simulink model "Spring_mass_damper_system"  (R2024a)
settings: Solver=VariableStepAuto  StartTime=0.0  StopTime=10  MaxStep=0.01  RelTol=1e-3
model workspace (MAT data in the model file):
  M = 10
  b = 50
  k = 100
settings Model: Creator=91839
settings SolverCC: AlgebraicLoopSolver=TrustRegion
settings DataIOCC: ExternalInput=data  LoadExternalInput=on  SaveFormat=Array  DSMLogging=off  ReturnWorkspaceOutputs=off
settings DebuggingCC: UnconnectedInputMsg=warning  UnconnectedOutputMsg=warning  UnconnectedLineMsg=warning
settings ModelReferenceCC: EnableRefExpFcnMdlSchedulingChecks=on
settings SFSimCC: CustomCodeUndefinedFunction=UseInterfaceOnly
settings RTWCC: GPUComputeCapability=3.5

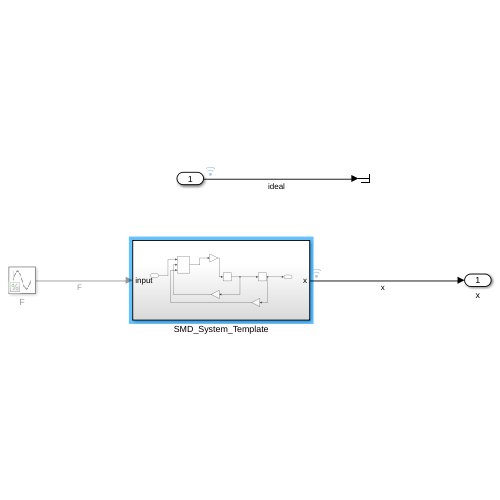
[thumbnail: Simulink's stored preview of the top-level diagram]
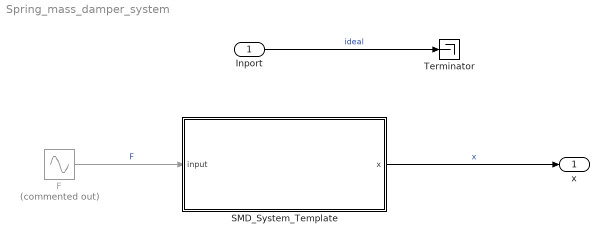
== system Spring_mass_damper_system ==
  Inport : Inport
  F : Sin  Commented=on  SampleTime=0
  SMD_System_Template : Subsystem
  Terminator : Terminator
  x : Outport
  wires:
  Inport/1 -> Terminator/1  "ideal"
  F/1 -> SMD_System_Template/1(input)  "F"
  SMD_System_Template/1(x) -> x/1  "x"

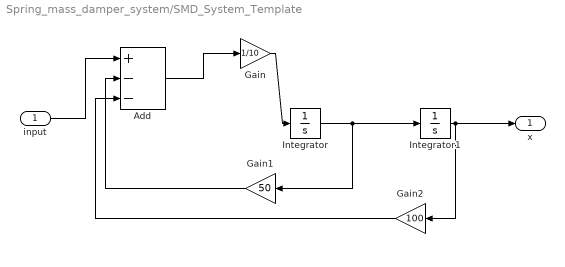
== system Spring_mass_damper_system/SMD_System_Template ==
  input : Inport
  Add : Sum  Inputs=+--
  Gain : Gain  Gain=1/10
  Gain1 : Gain  Gain=50
  Gain2 : Gain  Gain=100
  Integrator : Integrator
  Integrator1 : Integrator
  x : Outport
  wires:
  Integrator/1 -> Gain1/1, Integrator1/1
  Integrator1/1 -> Gain2/1, x/1
  input/1 -> Add/1
  Add/1 -> Gain/1
  Gain1/1 -> Add/2
  Gain2/1 -> Add/3
  Gain/1 -> Integrator/1
